simulink model "model2"  (R2023b)
settings: Solver=VariableStepAuto  StartTime=0.0  StopTime=10.0  RelTol=1e-3
values from neighbouring files (symbols this model uses):
  A = [0, 1, 0, 0 ... (first row only)    [e01.m]
  B = [0, 0 ... (first row only)    [e01.m]
  C = [1, 0, 0, 0 ... (first row only)    [e01.m]
  D = [0, 0 ... (first row only)    [e01.m]
  k = place(A,B,p)    [e01.m]
settings Model: Creator=Dell  LastModifiedBy=Dell

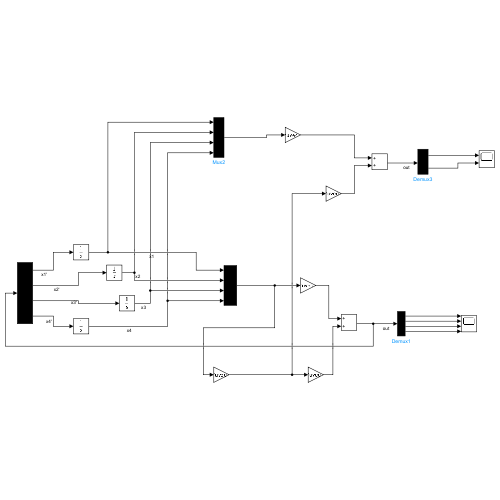
[thumbnail: Simulink's stored preview of the top-level diagram]
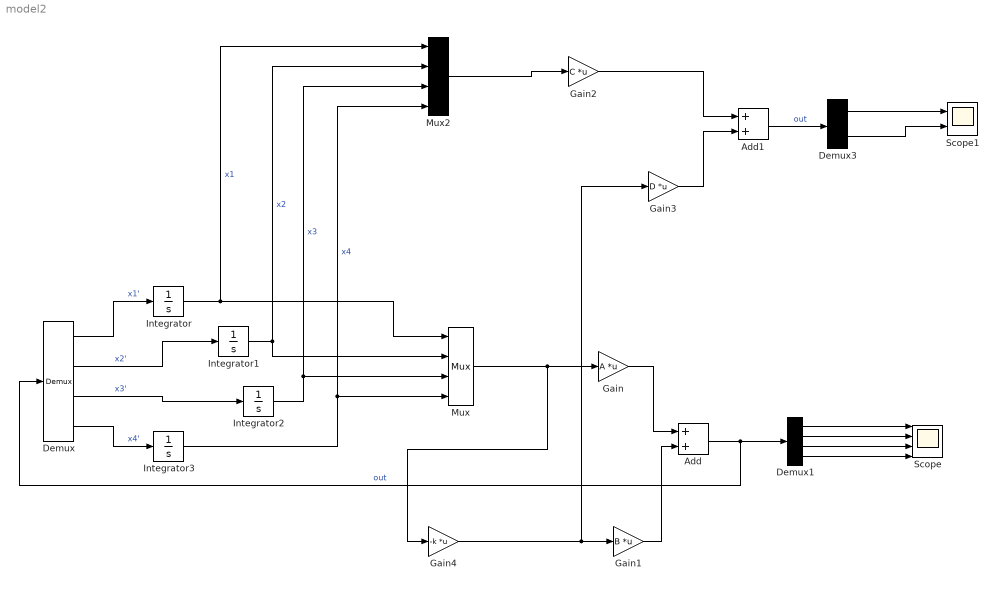
== system model2 ==
  Add : Sum
  Add1 : Sum
  Demux : Demux
  Demux1 : Demux
  Demux3 : Demux  Outputs=2
  Gain : Gain  Gain=A  Multiplication=Matrix(K*u) (u vector)
  Gain1 : Gain  Gain=B  Multiplication=Matrix(K*u) (u vector)
  Gain2 : Gain  Gain=C  Multiplication=Matrix(K*u) (u vector)
  Gain3 : Gain  Gain=D  Multiplication=Matrix(K*u) (u vector)
  Gain4 : Gain  Gain=-k  Multiplication=Matrix(K*u) (u vector)
  Integrator : Integrator  InitialCondition=10
  Integrator1 : Integrator  InitialCondition=20
  Integrator2 : Integrator  InitialCondition=-10
  Integrator3 : Integrator  InitialCondition=-20
  Mux : Mux
  Mux2 : Mux
  Scope : Scope  NumInputPorts=4
  Scope1 : Scope  NumInputPorts=2
  wires:
  Demux/1 -> Integrator/1  "x1'"
  Demux/2 -> Integrator1/1  "x2'"
  Demux/3 -> Integrator2/1  "x3'"
  Demux/4 -> Integrator3/1  "x4'"
  Integrator/1 -> Mux2/1, Mux/1  "x1"
  Integrator1/1 -> Mux/2, Mux2/2  "x2"
  Integrator2/1 -> Mux2/3, Mux/3  "x3"
  Integrator3/1 -> Mux2/4, Mux/4  "x4"
  Mux/1 -> Gain4/1, Gain/1
  Gain/1 -> Add/1
  Gain1/1 -> Add/2
  Add/1 -> Demux/1, Demux1/1  "out"
  Demux1/1 -> Scope/1
  Demux1/2 -> Scope/2
  Demux1/3 -> Scope/3
  Demux1/4 -> Scope/4
  Demux3/2 -> Scope1/2
  Demux3/1 -> Scope1/1
  Gain2/1 -> Add1/1
  Add1/1 -> Demux3/1  "out"
  Gain3/1 -> Add1/2
  Mux2/1 -> Gain2/1
  Gain4/1 -> Gain3/1, Gain1/1
